simulink model "Lab_06_Task02"  (R2015a)
settings: Solver=ode45  StartTime=0.0  StopTime=10.0  RelTol=1e-3
settings Model: Creator=Amir  LastModifiedBy=Amir

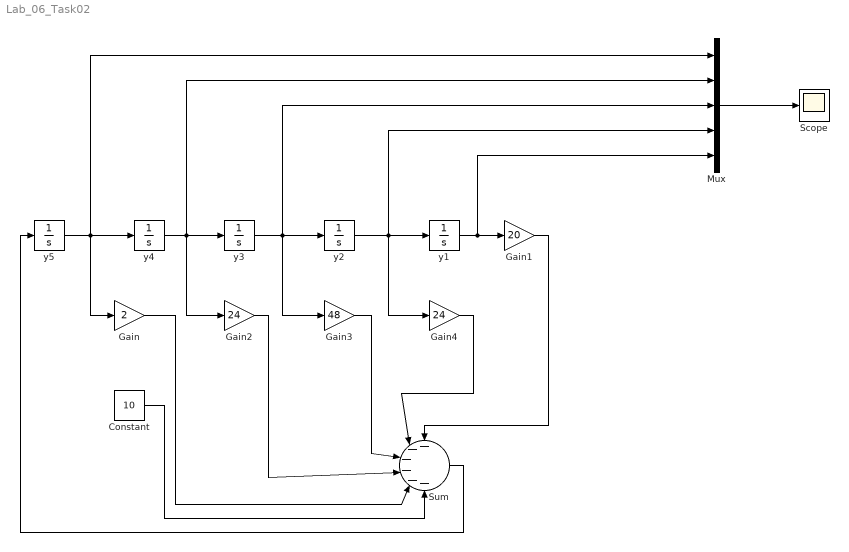
== system Lab_06_Task02 ==
  Constant : Constant  Value=10
  Gain : Gain  Gain=2
  Gain1 : Gain  Gain=20
  Gain2 : Gain  Gain=24
  Gain3 : Gain  Gain=48
  Gain4 : Gain  Gain=24
  Mux : Mux  Inputs=5
  Scope : Scope
  Sum : Sum  Inputs=------
  y1 : Integrator  InitialCondition=2
  y2 : Integrator  InitialCondition=5
  y3 : Integrator  InitialCondition=10
  y4 : Integrator  InitialCondition=-4
  y5 : Integrator  InitialCondition=-7
  wires:
  y5/1 -> Mux/1, Gain/1, y4/1
  y4/1 -> Mux/2, Gain2/1, y3/1
  y3/1 -> Mux/3, Gain3/1, y2/1
  y2/1 -> Mux/4, Gain4/1, y1/1
  y1/1 -> Mux/5, Gain1/1
  Gain1/1 -> Sum/1
  Gain4/1 -> Sum/2
  Gain3/1 -> Sum/3
  Gain2/1 -> Sum/4
  Gain/1 -> Sum/5
  Constant/1 -> Sum/6
  Sum/1 -> y5/1
  Mux/1 -> Scope/1
